simulink model "hil4DOFArmShared"  (R2017a)
settings: Solver=FixedStepAuto  StartTime=0.0  StopTime=inf  RelTol=1e-3
undefined symbols (not defined in the file): armDynamics, get, theta
libraries: vrlib x4, myo_lib x3, dspstat3 x2, sldrtlib x1
settings Model: Creator=ricardog  LastModifiedBy=ricardog
settings SolverCC: AutoInsertRateTranBlk=on

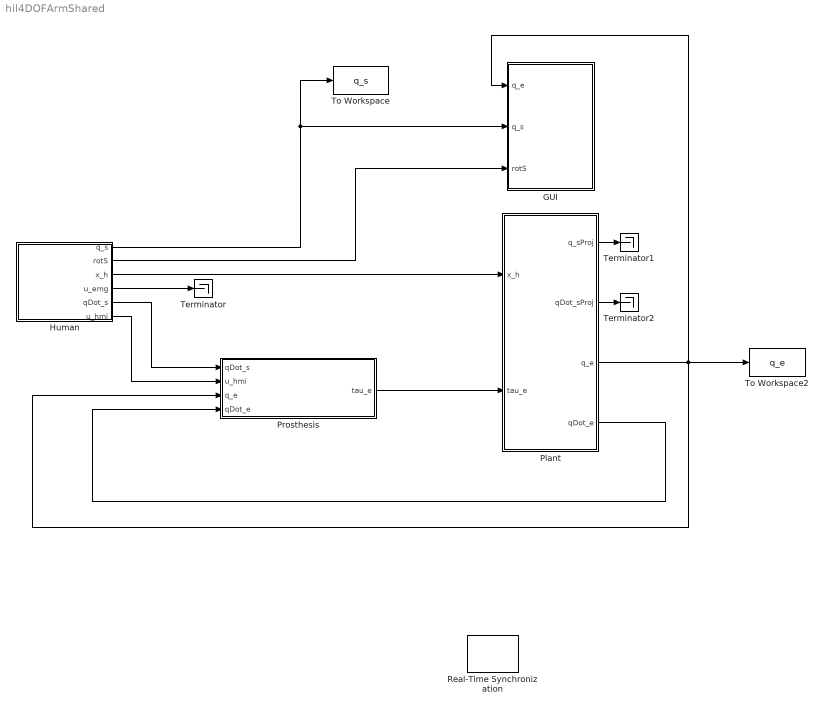
== system hil4DOFArmShared ==
  GUI : Subsystem
  Human : Subsystem
  Plant : Subsystem
  Prosthesis : Subsystem
  Real-Time Synchronization : sldrtlib/Real-Time Synchronization  SampleTime=0.01  MaxMissedTicks=50  ShowMissedTicks=off  YieldWhenWaiting=off
  Terminator : Terminator
  Terminator1 : Terminator
  Terminator2 : Terminator
  To Workspace : ToWorkspace  VariableName=q_s  SampleTime=-1
  To Workspace2 : ToWorkspace  VariableName=q_e  SampleTime=-1
  wires:
  Human/4(u_emg) -> Terminator/1
  Human/3(x_h) -> Plant/1(x_h)
  Plant/1(q_sProj) -> Terminator1/1
  Plant/2(qDot_sProj) -> Terminator2/1
  Human/1(q_s) -> To Workspace/1, GUI/2(q_s)
  Human/2(rotS) -> GUI/3(rotS)
  Plant/3(q_e) -> To Workspace2/1, Prosthesis/3(q_e), GUI/1(q_e)
  Plant/4(qDot_e) -> Prosthesis/4(qDot_e)
  Prosthesis/1(tau_e) -> Plant/2(tau_e)
  Human/5(qDot_s) -> Prosthesis/1(qDot_s)
  Human/6(u_hmi) -> Prosthesis/2(u_hmi)

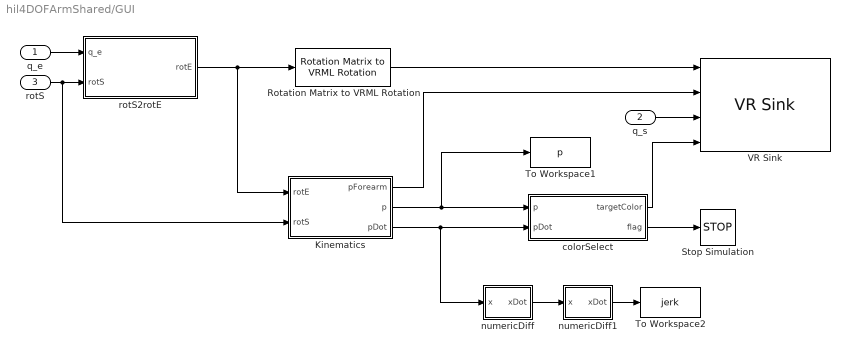
== system hil4DOFArmShared/GUI ==
  q_e : Inport
  q_s : Inport  Port=2
  rotS : Inport  Port=3
  Kinematics : Subsystem
  Rotation Matrix to VRML Rotation : vrlib/Utilities/Rotation Matrix to VRML Rotation  maxzero=1e-12
      settings: SourceProductName=Simulink 3D Animation  SourceProductBaseCode=VR
  Stop Simulation : Stop
  To Workspace1 : ToWorkspace  VariableName=p  SampleTime=-1
  To Workspace2 : ToWorkspace  VariableName=jerk  SampleTime=-1
  VR Sink : vrlib/VR Sink  InstantiateOnLoad=on  SampleTime=0.1  ViewEnable=on  RemoteChange=off  RemoteView=off  FieldsWritten=Forearm.rotation.4.1.1.double#Forearm.translation.3.1.1.double#UpperArm.rotation.4.1.1.double#EndTarget_material.diffuseColor.3.1.1.double  WorldFileName=C:\Users\ricardog\Documents\Workspace\HRSC_FW\GUI\armTargetsGUI.wrl  AutoView=on  VideoDimensions=[]  AllowVariableSize=off  FigureProperties="{'Position', 'Name', 'Viewpoint', 'CameraBound', 'CameraDirection', 'CameraPosition', 'CameraUpVector', 'ZoomFactor', 'Antialiasing', 'Headlight', 'Lighting', 'NavPanel', 'Sound', 'StatusBar', 'Stereo3D', 'Stereo3DCameraOffset', 'Stereo3DHIT', 'ToolBar', 'Textures', 'Transparency', 'Triad', 'Wireframe', 'NavZones', 'NavMode', 'NavSpeed', 'CaptureFileFormat', 'CaptureFileName', 'Record2DCompressMethod', 'Record2DCompressQuality', 'Record2D', 'Record2DFileName', 'Record2DFPS'; [7.5700000000000000e+02   1.3100000000000000e+02   7.6480000000000018e+02   5.7960000000000002e+02], '', 'FPV', 'on', [0.0000000000000000e+00   0.0000000000000000e+00  -1.0000000000000000e+00], [0.0000000000000000e+00   0.0000000000000000e+00   0.0000000000000000e+00], [0.0000000000000000e+00   1.0000000000000000e+00   0.0000000000000000e+00], [1.0000000000000000e+00], 'on', 'on', 'on', 'halfbar', 'on', 'on', 'off', [1.0000000149011612e-01], [0.0000000000000000e+00], 'on', 'on', 'on', 'none', 'off', 'off', 'examine', 'normal', 'tif', '%f_anim_%n.tif', 'auto', [7.5000000000000000e+01], 'off', '%f_anim_%n.avi', 'auto'}"
      settings: SourceProductBaseCode=VR
  colorSelect : MATLAB Function  TreatAsAtomicUnit=on
  numericDiff : Subsystem
  numericDiff1 : Subsystem
  rotS2rotE : MATLAB Function  TreatAsAtomicUnit=on
  wires:
  colorSelect/1(targetColor) -> VR Sink/4
  q_s/1 -> VR Sink/3
  Rotation Matrix to VRML Rotation/1 -> VR Sink/1
  rotS/1 -> rotS2rotE/2(rotS), Kinematics/2(rotS)
  rotS2rotE/1(rotE) -> Rotation Matrix to VRML Rotation/1, Kinematics/1(rotE)
  q_e/1 -> rotS2rotE/1(q_e)
  Kinematics/2(p) -> colorSelect/1(p), To Workspace1/1
  Kinematics/3(pDot) -> colorSelect/2(pDot), numericDiff/1(x)
  Kinematics/1(pForearm) -> VR Sink/2
  numericDiff/1(xDot) -> numericDiff1/1(x)
  numericDiff1/1(xDot) -> To Workspace2/1
  colorSelect/2(flag) -> Stop Simulation/1

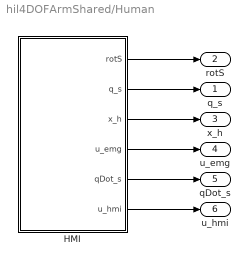
== system hil4DOFArmShared/Human ==
  HMI : Subsystem
  q_s : Outport
  rotS : Outport  Port=2
  x_h : Outport  Port=3
  u_emg : Outport  Port=4
  qDot_s : Outport  Port=5
  u_hmi : Outport  Port=6
  wires:
  HMI/1(rotS) -> rotS/1
  HMI/4(u_emg) -> u_emg/1
  HMI/3(x_h) -> x_h/1
  HMI/2(q_s) -> q_s/1
  HMI/5(qDot_s) -> qDot_s/1
  HMI/6(u_hmi) -> u_hmi/1

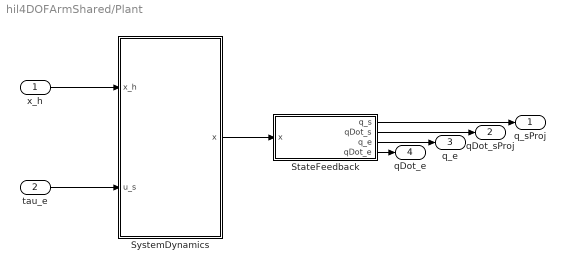
== system hil4DOFArmShared/Plant ==
  x_h : Inport
  tau_e : Inport  Port=2
  StateFeedback : Subsystem
  SystemDynamics : Subsystem
  q_sProj : Outport
  qDot_sProj : Outport  Port=2
  q_e : Outport  Port=3
  qDot_e : Outport  Port=4
  wires:
  SystemDynamics/1(x) -> StateFeedback/1(x)
  tau_e/1 -> SystemDynamics/2(u_s)
  StateFeedback/1(q_s) -> q_sProj/1
  StateFeedback/3(q_e) -> q_e/1
  StateFeedback/2(qDot_s) -> qDot_sProj/1
  StateFeedback/4(qDot_e) -> qDot_e/1
  x_h/1 -> SystemDynamics/1(x_h)

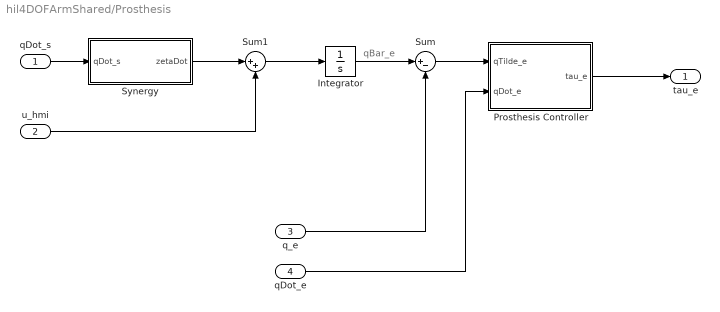
== system hil4DOFArmShared/Prosthesis ==
  note: qBar_e
  qDot_s : Inport
  u_hmi : Inport  Port=2
  q_e : Inport  Port=3
  qDot_e : Inport  Port=4
  Integrator : Integrator  InitialCondition=get(armDynamics,'qInit_e')
  Prosthesis Controller : Subsystem
  Sum : Sum  Inputs=|+-
  Sum1 : Sum  Inputs=|++
  Synergy : Subsystem
  tau_e : Outport
  wires:
  qDot_s/1 -> Synergy/1(qDot_s)
  Prosthesis Controller/1(tau_e) -> tau_e/1
  qDot_e/1 -> Prosthesis Controller/2(qDot_e)
  q_e/1 -> Sum/2
  Sum/1 -> Prosthesis Controller/1(qTilde_e)
  Integrator/1 -> Sum/1
  Synergy/1(zetaDot) -> Sum1/1
  Sum1/1 -> Integrator/1
  u_hmi/1 -> Sum1/2

== system hil4DOFArmShared/GUI/Kinematics ==
  rotE : Inport
  rotS : Inport  Port=2
  forwardKinematics : MATLAB Function  TreatAsAtomicUnit=on
  numericDiff : Subsystem
  pForearm : Outport
  p : Outport  Port=2
  pDot : Outport  Port=3
  wires:
  forwardKinematics/1(p) -> numericDiff/1(x), p/1
  forwardKinematics/2(pForearm) -> pForearm/1
  rotS/1 -> forwardKinematics/1(rotS)
  rotE/1 -> forwardKinematics/2(rotE)
  numericDiff/1(xDot) -> pDot/1

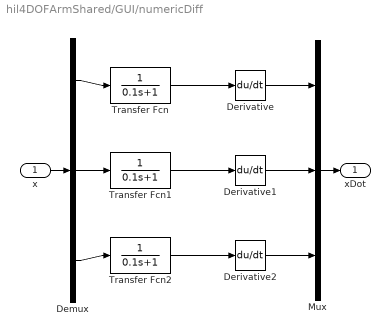
== system hil4DOFArmShared/GUI/numericDiff ==
  x : Inport
  Demux : Demux  Outputs=3
  Derivative : Derivative
  Derivative1 : Derivative
  Derivative2 : Derivative
  Mux : Mux  Inputs=3
  Transfer Fcn : TransferFcn  Denominator=[0.1 1]
  Transfer Fcn1 : TransferFcn  Denominator=[0.1 1]
  Transfer Fcn2 : TransferFcn  Denominator=[0.1 1]
  xDot : Outport
  wires:
  Mux/1 -> xDot/1
  Derivative1/1 -> Mux/2
  x/1 -> Demux/1
  Demux/3 -> Transfer Fcn2/1
  Derivative2/1 -> Mux/3
  Transfer Fcn/1 -> Derivative/1
  Demux/1 -> Transfer Fcn/1
  Derivative/1 -> Mux/1
  Transfer Fcn2/1 -> Derivative2/1
  Transfer Fcn1/1 -> Derivative1/1
  Demux/2 -> Transfer Fcn1/1

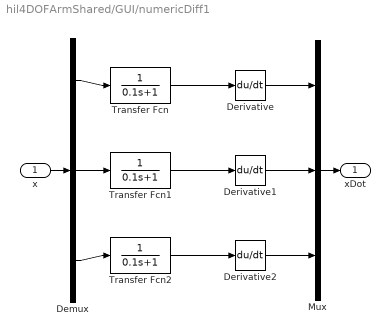
== system hil4DOFArmShared/GUI/numericDiff1 ==
  x : Inport
  Demux : Demux  Outputs=3
  Derivative : Derivative
  Derivative1 : Derivative
  Derivative2 : Derivative
  Mux : Mux  Inputs=3
  Transfer Fcn : TransferFcn  Denominator=[0.1 1]
  Transfer Fcn1 : TransferFcn  Denominator=[0.1 1]
  Transfer Fcn2 : TransferFcn  Denominator=[0.1 1]
  xDot : Outport
  wires:
  Mux/1 -> xDot/1
  Derivative1/1 -> Mux/2
  x/1 -> Demux/1
  Demux/3 -> Transfer Fcn2/1
  Derivative2/1 -> Mux/3
  Transfer Fcn/1 -> Derivative/1
  Demux/1 -> Transfer Fcn/1
  Derivative/1 -> Mux/1
  Transfer Fcn2/1 -> Derivative2/1
  Transfer Fcn1/1 -> Derivative1/1
  Demux/2 -> Transfer Fcn1/1

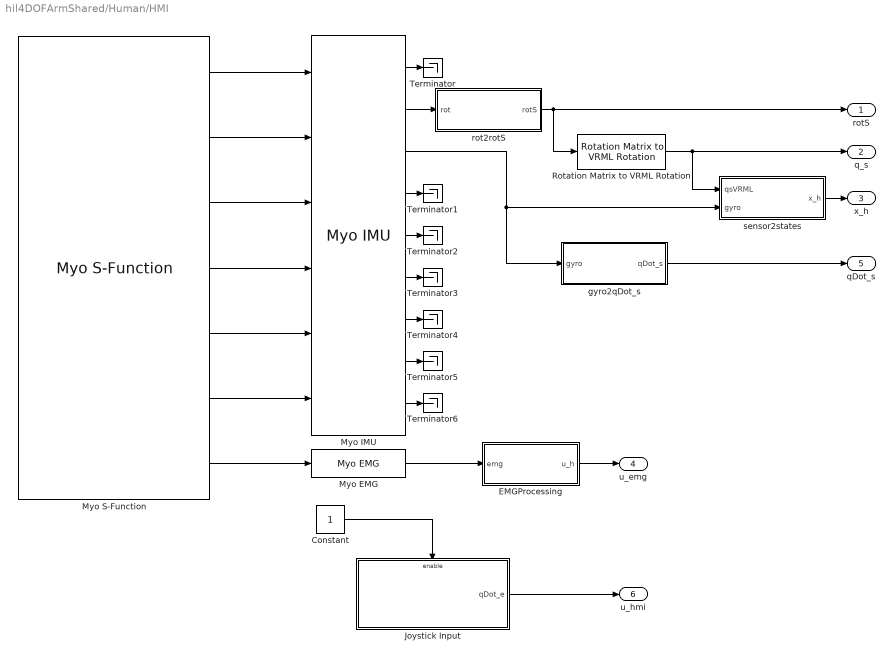
== system hil4DOFArmShared/Human/HMI ==
  Constant : Constant
  EMGProcessing : Subsystem
  Joystick Input : Subsystem
  Myo EMG : myo_lib/Myo EMG
  Myo IMU : myo_lib/Myo IMU
  Myo S-Function : myo_lib/Myo S-Function  emgEnabled=1  countMyos=1
  Rotation Matrix to VRML Rotation : vrlib/Utilities/Rotation Matrix to VRML Rotation  maxzero=1e-12
      settings: SourceProductName=Simulink 3D Animation  SourceProductBaseCode=VR
  Terminator{,1..6} (7 alike) : Terminator
  gyro2qDot_s : MATLAB Function  TreatAsAtomicUnit=on
  rot2rotS : MATLAB Function  TreatAsAtomicUnit=on
  sensor2states : MATLAB Function  TreatAsAtomicUnit=on
  rotS : Outport
  q_s : Outport  Port=2
  x_h : Outport  Port=3
  u_emg : Outport  Port=4
  qDot_s : Outport  Port=5
  u_hmi : Outport  Port=6
  wires:
  Myo S-Function/3 -> Myo IMU/3
  Myo S-Function/7 -> Myo EMG/1
  Myo S-Function/4 -> Myo IMU/4
  Myo S-Function/5 -> Myo IMU/5
  Myo S-Function/2 -> Myo IMU/2
  Myo S-Function/1 -> Myo IMU/1
  Myo S-Function/6 -> Myo IMU/6
  Myo EMG/1 -> EMGProcessing/1(emg)
  EMGProcessing/1(u_h) -> u_emg/1
  Myo IMU/3 -> gyro2qDot_s/1(gyro), sensor2states/2(gyro)
  Myo IMU/2 -> rot2rotS/1(rot)
  rot2rotS/1(rotS) -> rotS/1, Rotation Matrix to VRML Rotation/1
  Rotation Matrix to VRML Rotation/1 -> q_s/1, sensor2states/1(qsVRML)
  sensor2states/1(x_h) -> x_h/1
  gyro2qDot_s/1(qDot_s) -> qDot_s/1
  Myo IMU/1 -> Terminator/1
  Myo IMU/4 -> Terminator1/1
  Myo IMU/5 -> Terminator2/1
  Myo IMU/6 -> Terminator3/1
  Myo IMU/7 -> Terminator4/1
  Myo IMU/9 -> Terminator6/1
  Myo IMU/8 -> Terminator5/1
  Constant/1 -> Joystick Input/Enable
  Joystick Input/1(qDot_e) -> u_hmi/1

== system hil4DOFArmShared/Plant/StateFeedback ==
  x : Inport
  Demux : Demux
  q_s : Outport
  qDot_s : Outport  Port=2
  q_e : Outport  Port=3
  qDot_e : Outport  Port=4
  wires:
  x/1 -> Demux/1
  Demux/1 -> q_s/1
  Demux/3 -> qDot_s/1
  Demux/4 -> qDot_e/1
  Demux/2 -> q_e/1

== system hil4DOFArmShared/Plant/SystemDynamics ==
  x_h : Inport
  u_s : Inport  Port=2
  2DOFArm : MATLABSystem  System=armDynamics  kS=0  kE=0  dS=-1.2  dE=-1.2  lA=0.31  lF=0.34  mA=1.93  mF=1.52  q0=[ 0; pi/2 ]  qInit_s=pi/8  qInit_e=7*pi/8  qInit=[ pi/8; 7*pi/8 ]  qDotInit=[ 0; 0 ]  SimulateUsing=Code generation
      mask Type: armDynamics
      mask Display:
      | disp('armDynamics');
      | port_label('input',1,'x');
      | port_label('input',2,'u');
      | port_label('output',1,'xDot');
  Integrator : Integrator  InitialCondition=[get(armDynamics,'qInit');get(armDynamics,'qDotInit')]  UpperSaturationLimit=100  LowerSaturationLimit=-100
  States : Subsystem
  x : Outport
  wires:
  u_s/1 -> 2DOFArm/2
  2DOFArm/1 -> Integrator/1
  Integrator/1 -> States/1(xSim)
  x_h/1 -> States/2(x_h)
  States/1(x) -> 2DOFArm/1, x/1

== system hil4DOFArmShared/Prosthesis/Prosthesis Controller ==
  qTilde_e : Inport
  qDot_e : Inport  Port=2
  Kd : Gain  Gain=3
  Kp : Gain  Gain=50
  Sum : Sum  Inputs=|+-
  tau_e : Outport
  wires:
  qTilde_e/1 -> Kp/1
  qDot_e/1 -> Kd/1
  Kp/1 -> Sum/1
  Kd/1 -> Sum/2
  Sum/1 -> tau_e/1

== system hil4DOFArmShared/Prosthesis/Synergy ==
  qDot_s : Inport
  theta : Gain  Gain=theta  Multiplication=Matrix(K*u) (u vector)
  zetaDot : Outport
  wires:
  theta/1 -> zetaDot/1
  qDot_s/1 -> theta/1

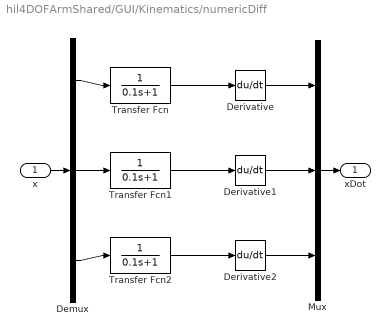
== system hil4DOFArmShared/GUI/Kinematics/numericDiff ==
  x : Inport
  Demux : Demux  Outputs=3
  Derivative : Derivative
  Derivative1 : Derivative
  Derivative2 : Derivative
  Mux : Mux  Inputs=3
  Transfer Fcn : TransferFcn  Denominator=[0.1 1]
  Transfer Fcn1 : TransferFcn  Denominator=[0.1 1]
  Transfer Fcn2 : TransferFcn  Denominator=[0.1 1]
  xDot : Outport
  wires:
  Mux/1 -> xDot/1
  Derivative1/1 -> Mux/2
  x/1 -> Demux/1
  Demux/3 -> Transfer Fcn2/1
  Derivative2/1 -> Mux/3
  Transfer Fcn/1 -> Derivative/1
  Demux/1 -> Transfer Fcn/1
  Derivative/1 -> Mux/1
  Transfer Fcn2/1 -> Derivative2/1
  Transfer Fcn1/1 -> Derivative1/1
  Demux/2 -> Transfer Fcn1/1

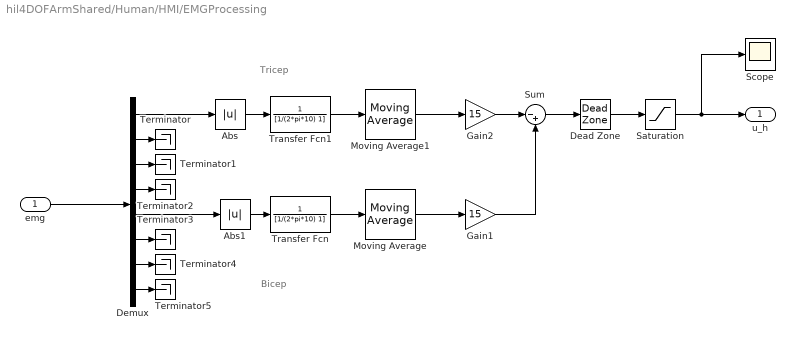
== system hil4DOFArmShared/Human/HMI/EMGProcessing ==
  note: Tricep
  note: Bicep
  emg : Inport
  Abs : Abs
  Abs1 : Abs
  Dead Zone : DeadZone  LowerValue=-0.7  UpperValue=0.7  SaturateOnIntegerOverflow=on
  Demux : Demux  Outputs=8
  Gain1 : Gain  Gain=15
  Gain2 : Gain  Gain=15
  Moving Average : dspstat3/Moving Average  Method=Sliding window  SpecifyWindowLength=on  WindowLength=1000  ForgettingFactor=0.9  SimulateUsing=Code generation
  Moving Average1 : dspstat3/Moving Average  Method=Sliding window  SpecifyWindowLength=on  WindowLength=1000  ForgettingFactor=0.9  SimulateUsing=Code generation
  Saturation : Saturate  UpperLimit=3  LowerLimit=-3
  Scope : Scope
  Sum : Sum  Inputs=|-+
  Terminator{,1..5} (6 alike) : Terminator
  Transfer Fcn : TransferFcn  Denominator=[1/(2*pi*10) 1]
  Transfer Fcn1 : TransferFcn  Denominator=[1/(2*pi*10) 1]
  u_h : Outport
  wires:
  Transfer Fcn/1 -> Moving Average/1
  Moving Average/1 -> Gain1/1
  Moving Average1/1 -> Gain2/1
  Demux/5 -> Abs1/1
  Demux/1 -> Abs/1
  Abs1/1 -> Transfer Fcn/1
  Transfer Fcn1/1 -> Moving Average1/1
  Abs/1 -> Transfer Fcn1/1
  emg/1 -> Demux/1
  Gain1/1 -> Sum/2
  Gain2/1 -> Sum/1
  Saturation/1 -> Scope/1, u_h/1
  Sum/1 -> Dead Zone/1
  Dead Zone/1 -> Saturation/1
  Demux/2 -> Terminator/1
  Demux/3 -> Terminator1/1
  Demux/4 -> Terminator2/1
  Demux/6 -> Terminator3/1
  Demux/7 -> Terminator4/1
  Demux/8 -> Terminator5/1

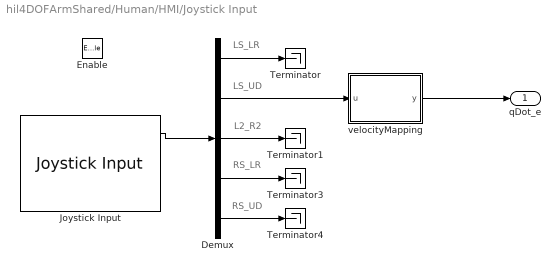
== system hil4DOFArmShared/Human/HMI/Joystick Input ==
  note: RS_UD
  note: RS_LR
  note: L2_R2
  note: LS_UD
  note: LS_LR
  Enable : EnablePort
  Demux : Demux  Outputs=5
  Joystick Input : vrlib/Joystick Input  joyid=1  adjustports=on  forcefeed=off
      settings: SourceProductBaseCode=VR
  Terminator{,1,3..4} (4 alike) : Terminator
  velocityMapping : MATLAB Function  TreatAsAtomicUnit=on
  qDot_e : Outport
  wires:
  Joystick Input/1 -> Demux/1
  Demux/3 -> Terminator1/1
  Demux/1 -> Terminator/1
  Demux/2 -> velocityMapping/1(u)
  Demux/4 -> Terminator3/1
  Demux/5 -> Terminator4/1
  velocityMapping/1(y) -> qDot_e/1

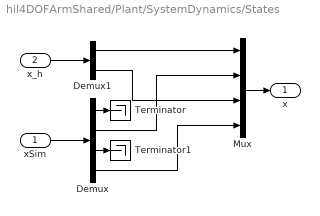
== system hil4DOFArmShared/Plant/SystemDynamics/States ==
  xSim : Inport
  x_h : Inport  Port=2
  Demux : Demux
  Demux1 : Demux  Outputs=2
  Mux : Mux
  Terminator : Terminator
  Terminator1 : Terminator
  x : Outport
  wires:
  xSim/1 -> Demux/1
  x_h/1 -> Demux1/1
  Mux/1 -> x/1
  Demux1/1 -> Mux/1
  Demux1/2 -> Mux/3
  Demux/2 -> Mux/2
  Demux/4 -> Mux/4
  Demux/1 -> Terminator/1
  Demux/3 -> Terminator1/1

== matlab function hil4DOFArmShared/GUI/colorSelect ==
  data: p input; targetColor output; pDot input; flag output
function [targetColor, flag] = colorSelect(p,pDot)
p_f = [0.5969;-0.0670;-0.2];   % Desired end position
pNorm = norm(p-p_f);
pDotNorm = norm(pDot);
if(pNorm<0.03 && pDotNorm<0.02)
    R = 0;
    G = 1;
    B = 0;
    flag = 1;
elseif(pNorm<0.03 && pDotNorm<0.05)
    R = 0;
    G = 1;
    B = 0;
    flag = 0;
else
    R = 0;
    G = 0;
    B = 1;
    flag = 0;
end
targetColor = [R;G;B];

== matlab function hil4DOFArmShared/Human/HMI/gyro2qDot_s ==
  data: gyro input; qDot_s output
% rot2rotS Converts fixed sensor frame sensor rotation matrix to VRML fixed
% frame.
% @in gyro gyroscope angular velocity vector.
% @out qDot_s shoulder angular velocity vector.
%
% Change log:
% Date        |   Comment           |     Owner
%-------------------------------------------------------
% 06/09/2017  | Creation            |     ricardog
% dd/mm/yyyy  | xxxxxxxxxxxxxxxx    |     xxxxxxxx
%
function qDot_s = gyro2qDot_s(gyro)
qDot_s = [1,-1,1].*deg2rad([gyro(3),gyro(2),gyro(1)]);

== matlab function hil4DOFArmShared/Human/HMI/sensor2states ==
  data: qsVRML input; gyro input; x_h output
% gyro2qsProjDot Converts sensor angular position and velocity data into
% states states for the dynamic model. States:
% qsProj shoulder angular position projection into the direction of elbow
% joint.
% qsProjDot shoulder angular velocity projection in the direction of elbow
% joint.
% @in qsVRML shoulder angular position vector in VRML representation.
% @in gyro gyroscope angular velocity vector.
% @out x_h equivalent arm model state projections.
%
% Change log:
% Date        |   Comment           |     Owner
%-------------------------------------------------------
% 06/09/2017  | Creation            |     ricardog
% dd/mm/yyyy  | xxxxxxxxxxxxxxxx    |     xxxxxxxx
%
function x_h = sensor2states(qsVRML,gyro)

x_h = [qsVRML(1)*qsVRML(4);
       -deg2rad(gyro(2))];

== matlab function hil4DOFArmShared/Human/HMI/rot2rotS ==
  data: rot input; rotS output
% rot2rotS Converts fixed sensor frame sensor rotation matrix to VRML fixed
% frame.
% @in rot fixed sensor frame sensor rotation matrix.
% @out rotS VRML fixed frame shoulder rotation matrix.
%
% Change log:
% Date        |   Comment           |     Owner
%-------------------------------------------------------
% 06/09/2017  | Creation            |     ricardog
% dd/mm/yyyy  | xxxxxxxxxxxxxxxx    |     xxxxxxxx
%
function rotS = rot2rotS(rot)
% Fixed sensor frame -90deg x rotation, fixed sensor frame rotation
% converts to VRML fixed frame. VRML fixed frame 90deg z rotation converts
% to shoulder zero frame.
rotS = rotx(-90)*rot*rotz(90)*roty(-90);

== matlab function hil4DOFArmShared/GUI/Kinematics/forwardKinematics ==
  data: rotS input; p output; rotE input; pForearm output
%
%
function [p,pForearm] = forwardKinematics(rotS,rotE)
% Get arm length
lA = get(armDynamics,'lA');
lF = get(armDynamics,'lF');
% Create distance vectors in local frame
rOA = [0;-lA;0];
rAF = [0;-lF;0];
rAGF = [0;-lF/2;0];
pOA = rotS*rOA;
% Hand position
p = pOA+rotE*rAF;
% Forearm centre of mass position (middle)
pForearm = pOA+rotE*rAGF;

== matlab function hil4DOFArmShared/GUI/rotS2rotE ==
  data: q_e input; rotS input; rotE output
% rotS2rotE Converts elbow rotation into VRML fixed frame rotation matrix.
% @in q_e elbow joint angle in radians.
% @in rotS VRML fixed frame shoulder rotation matrix.
% @out rotE VRML fixed frame elbow rottation matrix.
%
% Change log:
% Date        |   Comment           |     Owner
%-------------------------------------------------------
% 06/09/2017  | Creation            |     ricardog
% dd/mm/yyyy  | xxxxxxxxxxxxxxxx    |     xxxxxxxx
%
function rotE = rotS2rotE(q_e,rotS)
rotE = rotS*rotz(rad2deg(q_e));

== matlab function hil4DOFArmShared/Human/HMI/Joystick Input/velocityMapping ==
  data: u input; y output
function y = inputMod(u)
% Modifies input to fit model and rounds to certain decimal points.
% Change precision by modifying variable pres. Application dependent.
pres = 100000;
maxVel = 0.5;
y = round(pres*maxVel*u)/pres;
end
